simulink model "Pontoinicio"  (R2012b)
settings: Solver=ode1  StartTime=0.0  StopTime=5  FixedStep=0.05  RelTol=1e-3
libraries: opclib x2
settings Model: Creator=Leonardo  LastModifiedBy=Josias
settings DataIOCC: SignalLoggingSaveFormat=ModelDataLogs
settings OptimizationCC: ExpressionDepthLimit=128
settings DebuggingCC: UnderspecifiedInitializationDetection=Simplified  MultiTaskDSMMsg=warning  MultiTaskCondExecSysMsg=none  StateNameClashWarn=none  StrictBusMsg=None
settings RTWCC: IncludeERTFirstTime=on
settings CodeAppCC: CustomSymbolStrType=$N$R$M_T  InternalIdentifier=Shortened
settings GRTTargetCC: CodeReplacementLibrary=None  CPPClassGenCompliant=on

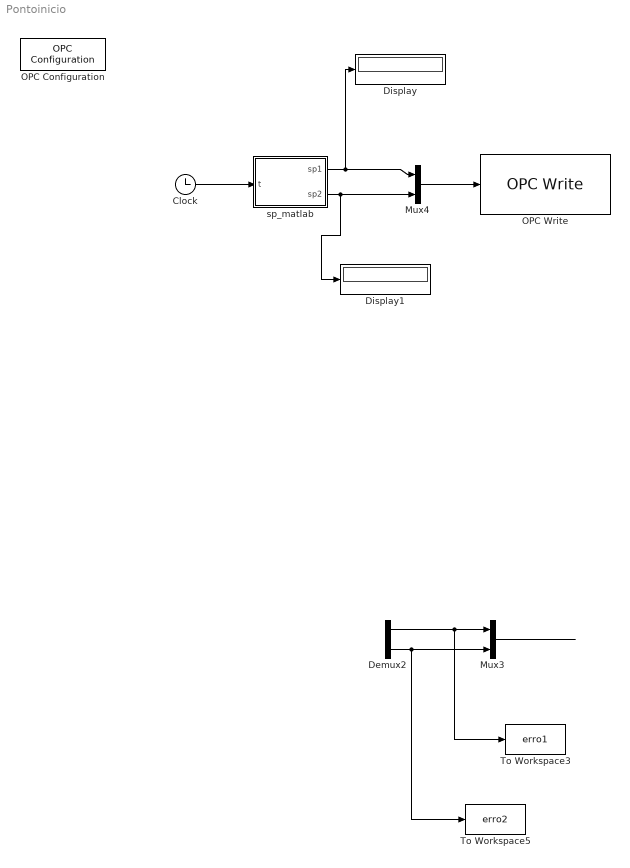
== system Pontoinicio ==
  Clock : Clock
  Demux2 : Demux  Outputs=2
  Display : Display
  Display1 : Display
  Mux3 : Mux  Inputs=2
  Mux4 : Mux  Inputs=2
  OPC Configuration : opclib/OPC Configuration  opcServers=localhost/ElipseSCADA.OPCSvr.1/10  errMissingItems=Error  errReadWrite=Warn  errShutdown=Error  errRTViolation=Warn  rtEnable=on  speedup=1  showLatency=off  beingUsed=on
  OPC Write : opclib/OPC Write  serverHost=localhost  serverID=ElipseSCADA.OPCSvr.1  itemIDs=Tags.setpoint_teta_1, Tags.setpoint_teta_2  writeMode=Synchronous  updateRate=0
  To Workspace3 : ToWorkspace  VariableName=erro1  SampleTime=-1
  To Workspace5 : ToWorkspace  VariableName=erro2  SampleTime=-1
  sp_matlab : MATLAB Function  TreatAsAtomicUnit=on
  wires:
  Demux2/2 -> To Workspace5/1, Mux3/2
  Demux2/1 -> To Workspace3/1, Mux3/1
  ? -> Demux2/1
  Mux3/1 -> ?
  Mux4/1 -> OPC Write/1
  sp_matlab/2(sp2) -> Display1/1, Mux4/2
  sp_matlab/1(sp1) -> Display/1, Mux4/1
  Clock/1 -> sp_matlab/1(t)

== matlab function Pontoinicio/sp_matlab ==
  data: sp1 output; t input; sp2 output
function [sp1, sp2] = fcn(t)

sp1 = 1686;
sp2 = 1097;

y =[sp1 sp2];
